simulink library "lic"  (R2021b)
settings: Solver=VariableStepAuto  StartTime=0.0  StopTime=10.0  RelTol=1e-3
undefined symbols (not defined in the file or in its folder): C_TICK_TIME_S, ENUM_LANEQUALITY_HIGH, ENUM_LANEQUALITY_MEDIUM, ENUM_LFCSTATE_DEGRADED, FALSE, KAPP_VehicleWidth_m, KLIC_C0CrossingThr_m, KLIC_C1Max4Act_rad, KLIC_C2Max4Act_rat, KLIC_C2Max4Disable_rat, KLIC_C2Max4DisableThr_s, KLIC_CalDefaultTLC_s, KLIC_CalTLCMax_s, KLIC_CalTLCMin_s, KLIC_DefaultLaneWidth_m, KLIC_Lane4ActThr_s, KLIC_LANEQUALITY_rat, KLIC_LANEQUALITYHysis_rat, KLIC_LaneWidHoldOnTime_s, KLIC_LaneWidRampFinErrThres_m, KLIC_LaneWidRampFinTimeThres_s, KLIC_LaneWidRampInFalRt_mps, KLIC_LaneWidRampInRisRt_mps, KLIC_LaneWidRampOutFalRt_mps, KLIC_LaneWidRampOutRisRt_mps, KLIC_LaneWidthLowThr_m, KLIC_LaneWidthUpThr_m, KLIC_TLCTriggerThrHysis_s, MLIC_TLCThr4LKA_s, TRUE
libraries: adcu_lib x20, simulink x14
(part 3 of 3)

== system lic/LIC/lic/LaneCalculation/UsingRawLaneL/Subsystem ==
  UsingRawLaneL_flg : Inport
  VISD_LaneC0L_m : Inport  Port=2
  VLIC_EstLaneC0L_m : Inport  Port=3
  VISD_LaneC1L_rad : Inport  Port=4
  VLIC_EstLaneC1L_rad : Inport  Port=5
  VISD_LaneC2L_rat : Inport  Port=6
  VLIC_EstLaneC2L_rat : Inport  Port=7
  VISD_LaneC3L_rat : Inport  Port=8
  VLIC_EstLaneC3L_rat : Inport  Port=9
  VISD_ViewRangeEndL_m : Inport  Port=10
  VLIC_EstViewRangeEndL_m : Inport  Port=11
  Switch{1,4..7} (5 alike) : Switch  Criteria=u2 ~= 0
  OptLaneC0L : Outport
  OptLaneC1L : Outport  Port=2
  OptLaneC2L : Outport  Port=3
  OptLaneC3L : Outport  Port=4
  OptViewRange_L : Outport  Port=5
  wires:
  Switch1/1 -> OptViewRange_L/1  "OptViewRange_L"
  VLIC_EstViewRangeEndL_m/1 -> Switch1/3
  UsingRawLaneL_flg/1 -> Switch5/2, Switch1/2, Switch7/2, Switch6/2, Switch4/2
  VISD_ViewRangeEndL_m/1 -> Switch1/1
  Switch5/1 -> OptLaneC1L/1  "OptLaneC1L"
  Switch4/1 -> OptLaneC0L/1  "OptLaneC0L"
  Switch7/1 -> OptLaneC3L/1  "OptLaneC3L"
  VLIC_EstLaneC3L_rat/1 -> Switch7/3
  VISD_LaneC3L_rat/1 -> Switch7/1
  Switch6/1 -> OptLaneC2L/1  "OptLaneC2L"
  VLIC_EstLaneC2L_rat/1 -> Switch6/3
  VISD_LaneC2L_rat/1 -> Switch6/1
  VLIC_EstLaneC1L_rad/1 -> Switch5/3
  VISD_LaneC1L_rad/1 -> Switch5/1
  VLIC_EstLaneC0L_m/1 -> Switch4/3
  VISD_LaneC0L_m/1 -> Switch4/1

== system lic/LIC/lic/LaneCalculation/UsingRawLaneR/Subsystem ==
  UsingRawLaneR_flg : Inport
  VISD_LaneC0R_m : Inport  Port=2
  VLIC_EstLaneC0R_m : Inport  Port=3
  VISD_LaneC1R_rad : Inport  Port=4
  VLIC_EstLaneC1R_rad : Inport  Port=5
  VISD_LaneC2R_rat : Inport  Port=6
  VLIC_EstLaneC2R_rat : Inport  Port=7
  VISD_LaneC3R_rat : Inport  Port=8
  VLIC_EstLaneC3R_rat : Inport  Port=9
  VISD_ViewRangeEndR_m : Inport  Port=10
  VLIC_EstViewRangeEndR_m : Inport  Port=11
  Switch{1,4..7} (5 alike) : Switch  Criteria=u2 ~= 0
  OptLaneC0R : Outport
  OptLaneC1R : Outport  Port=2
  OptLaneC2R : Outport  Port=3
  OptLaneC3R : Outport  Port=4
  OptViewRange_R : Outport  Port=5
  wires:
  Switch1/1 -> OptViewRange_R/1  "OptViewRange_R"
  VLIC_EstViewRangeEndR_m/1 -> Switch1/3
  UsingRawLaneR_flg/1 -> Switch5/2, Switch1/2, Switch7/2, Switch6/2, Switch4/2
  VISD_ViewRangeEndR_m/1 -> Switch1/1
  Switch5/1 -> OptLaneC1R/1  "OptLaneC1R"
  Switch4/1 -> OptLaneC0R/1  "OptLaneC0R"
  Switch7/1 -> OptLaneC3R/1  "OptLaneC3R"
  VLIC_EstLaneC3R_rat/1 -> Switch7/3
  VISD_LaneC3R_rat/1 -> Switch7/1
  Switch6/1 -> OptLaneC2R/1  "OptLaneC2R"
  VLIC_EstLaneC2R_rat/1 -> Switch6/3
  VISD_LaneC2R_rat/1 -> Switch6/1
  VLIC_EstLaneC1R_rad/1 -> Switch5/3
  VISD_LaneC1R_rad/1 -> Switch5/1
  VLIC_EstLaneC0R_m/1 -> Switch4/3
  VISD_LaneC0R_m/1 -> Switch4/1

== stateflow chart lic/LIC/lic/LaneCalculation/C1L_Bias/Forgetting_factor/FF ==
  state Forget_Factor
    (default) -> (junction 10) : {P=1;
        | C1LBias_new_store = C1LBias_new;
        | P_L = P;
        | C1L_Bias = C1LBias_new_store;}
    Forget_Factor -> (junction 10)
    (junction 10) -> (junction 13) : {C1LBias_new_store = C1LBias_new_store + P*(C1LBias_new - C1LBias_new_store)/(Forget_Factor+P);
        | P = (P-P*P/(Forget_Factor+P))/Forget_Factor;
        | P_L=P;
        | C1L_Bias=C1LBias_new_store;}
  data: C1LBias_new input; P local single; C1LBias_new_store local single; Forget_Factor input; C1L_Bias output single; P_L output single

== stateflow chart lic/LIC/lic/LaneCalculation/Lane_status ==
  (default) -> (junction 9)
  (junction 9) -> (junction 10) [order 1] : [VLIC_LeftLaneAvail_fig && VLIC_RightLaneAvail_fig]
  (junction 9) -> (junction 16) [order 2]
  (junction 10) -> (junction 12) : {SWCase=1;
      | LR_avail=TRUE;
      | R_avail=FALSE;
      | L_avail=FALSE;
      | NO_avail=FALSE;}
  (junction 16) -> (junction 18) [order 1] : [(!VLIC_C2Diff_flg || !VLIC_LeftLaneAvail_fig) && VLIC_RightLaneAvail_fig]
  (junction 16) -> (junction 22) [order 2]
  (junction 18) -> (junction 20) : {SWCase=2;
      | LR_avail=FALSE;
      | R_avail=TRUE;
      | L_avail=FALSE;
      | NO_avail=FALSE;}
  (junction 22) -> (junction 24) [order 1] : [VLIC_LeftLaneAvail_fig && (VLIC_C2Diff_flg || !VLIC_RightLaneAvail_fig)]
  (junction 22) -> (junction 34) [order 2] : {SWCase=4;
      | LR_avail=FALSE;
      | R_avail=FALSE;
      | L_avail=FALSE;
      | NO_avail=TRUE;}
  (junction 24) -> (junction 26) : {SWCase=3;
      | LR_avail=FALSE;
      | R_avail=FALSE;
      | L_avail=TRUE;
      | NO_avail=FALSE;}
  (junction 26) -> (junction 34)
  (junction 20) -> (junction 26)
  (junction 12) -> (junction 20)
  data: VLIC_LeftLaneAvail_fig input; VLIC_RightLaneAvail_fig input; SWCase output single; LR_avail output boolean; R_avail output boolean; L_avail output boolean; NO_avail output boolean; TRUE parameter; FALSE parameter; VLIC_C2Diff_flg input

== stateflow chart lic/LIC/lic/LaneCalculation/C1R_Bias/Forgetting_factor/FF ==
  state Forget_Factor
    (default) -> (junction 10) : {P=1;
        | C1RBias_new_store = C1RBias_new;
        | P_R = P;
        | C1R_Bias = C1RBias_new_store;}
    Forget_Factor -> (junction 10)
    (junction 10) -> (junction 13) : {C1RBias_new_store = C1RBias_new_store + P*(C1RBias_new - C1RBias_new_store)/(Forget_Factor+P);
        | P = (P-P*P/(Forget_Factor+P))/Forget_Factor;
        | P_R=P;
        | C1R_Bias=C1RBias_new_store;}
  data: C1RBias_new input; P local single; C1RBias_new_store local single; Forget_Factor input; C1R_Bias output single; P_R output single

== stateflow chart lic/LIC/lic/LaneCalculation/LaneProcess/Chart ==
  (default) -> (junction 21)
  (junction 21) -> (junction 22) [order 1] : [VINP_LnMk1Side_enum == ENUM_LnMk1Side_Left && VINP_LnMk2Side_enum == ENUM_LnMk2Side_Right]
  (junction 21) -> (junction 23) [order 2]
  (junction 22) -> (junction 27) : {VLIC_HLC0L_m=VINP_Ln1C0_m;
      | VLIC_HLC1L_rad=VINP_Ln1C1_rad;
      | VLIC_HLC2L_1pm=VINP_Ln1C2_1pm;
      | VLIC_HLC3L_1pmm=VINP_Ln1C3_1pmm;
      | VLIC_HLQualityL_rat=VINP_LnMk1Cnfdnce_rat;
      | VLIC_HLViewRangeL_m=VINP_LnMk1EndVR_m-VINP_LnMk1StartVR_m;
      | VLIC_HLC0R_m=VINP_Ln2C0_m;
      | VLIC_HLC1R_rad=VINP_Ln2C1_rad;
      | VLIC_HLC2R_1pm=VINP_Ln2C2_1pm;
      | VLIC_HLC3R_1pmm=VINP_Ln2C3_1pmm;
      | VLIC_HLQualityR_rat=VINP_LnMk2Cnfdnce_rat;
      | VLIC_HLViewRangeR_m=VINP_LnMk2EndVR_m-VINP_LnMk2StartVR_m;}
  (junction 23) -> (junction 24) [order 1] : [VINP_LnMk1Side_enum==ENUM_LnMk1Side_Right && VINP_LnMk2Side_enum == ENUM_LnMk2Side_Left]
  (junction 23) -> (junction 25) [order 2] : {VLIC_HLC0L_m=ZERO_INT;
      | VLIC_HLC1L_rad=ZERO_INT;
      | VLIC_HLC2L_1pm=ZERO_INT;
      | VLIC_HLC3L_1pmm=ZERO_INT;
      | VLIC_HLQualityL_rat=ZERO_INT;
      | VLIC_HLViewRangeL_m=ZERO_INT;
      | VLIC_HLC0R_m=ZERO_INT;
      | VLIC_HLC1R_rad=ZERO_INT;
      | VLIC_HLC2R_1pm=ZERO_INT;
      | VLIC_HLC3R_1pmm=ZERO_INT;
      | VLIC_HLQualityR_rat=ZERO_INT;
      | VLIC_HLViewRangeR_m=ZERO_INT;}
  (junction 24) -> (junction 26) : {VLIC_HLC0L_m=VINP_Ln2C0_m;
      | VLIC_HLC1L_rad=VINP_Ln2C1_rad;
      | VLIC_HLC2L_1pm=VINP_Ln2C2_1pm;
      | VLIC_HLC3L_1pmm=VINP_Ln2C3_1pmm;
      | VLIC_HLQualityL_rat=VINP_LnMk2Cnfdnce_rat;
      | VLIC_HLViewRangeL_m=VINP_LnMk2EndVR_m-VINP_LnMk2StartVR_m;
      | VLIC_HLC0R_m=VINP_Ln1C0_m;
      | VLIC_HLC1R_rad=VINP_Ln1C1_rad;
      | VLIC_HLC2R_1pm=VINP_Ln1C2_1pm;
      | VLIC_HLC3R_1pmm=VINP_Ln1C3_1pmm;
      | VLIC_HLQualityR_rat=VINP_LnMk1Cnfdnce_rat;
      | VLIC_HLViewRangeR_m=VINP_LnMk1EndVR_m-VINP_LnMk1StartVR_m;}
  (junction 26) -> (junction 25)
  (junction 27) -> (junction 26)
  (junction 25) -> (junction 28)
  data: VINP_LnMk1Side_enum input; VINP_LnMk2Side_enum input; VINP_Ln1C0_m input; VINP_Ln1C1_rad input; VINP_Ln1C2_1pm input; VINP_Ln1C3_1pmm input; VINP_Ln2C0_m input; VINP_Ln2C1_rad input; VINP_Ln2C2_1pm input; VINP_Ln2C3_1pmm input; VLIC_HLC0L_m output; VLIC_HLC1L_rad output; VLIC_HLC2L_1pm output; VLIC_HLC3L_1pmm output; VLIC_HLC0R_m output; VLIC_HLC1R_rad output; VLIC_HLC2R_1pm output; VLIC_HLC3R_1pmm output; VINP_LnMk1Cnfdnce_rad input; VINP_LnMk2Cnfdnce_rad input; VINP_LnMk1StartVR_m input; VINP_LnMk1EndVR_m input; VINP_LnMk2StartVR_m input; VINP_LnMk2EndVR_m input; VLIC_HLViewRangeL_m output; VLIC_HLViewRangeR_m output; VLIC_HLQualityL_rat output; VLIC_HLQualityR_rat output
